simulink subsystem "Driver_Input"  (R2021b)
settings: Solver=VariableStepAuto  StartTime=0.0  StopTime=10.0  RelTol=1e-3
PostLoadFcn:
  | if any(exist('dsrtsu_mdlpostloadfcn', 'file') ~= 0), dsrtsu_mdlpostloadfcn('Execute', bdroot); end
libraries: simulink x9, dspstat3 x7, rtican x3, rti1401lib_adc_type4 x1
(part 2 of 2)

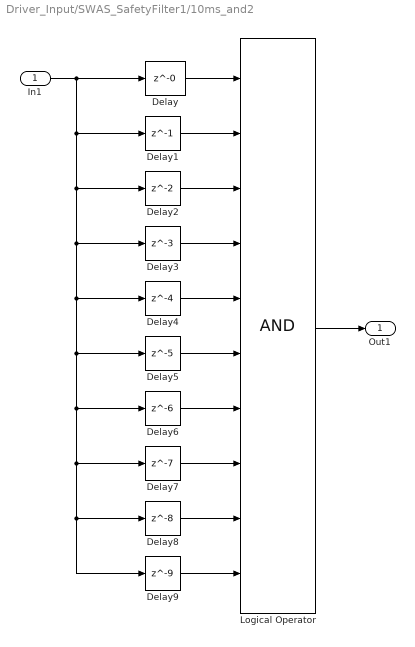
== system Driver_Input/SWAS_SafetyFilter1/10ms_and2 ==
  In1 : Inport
  Delay : Delay  DelayLength=0  InitialCondition=0
  Delay1 : Delay  DelayLength=1  InitialCondition=0
  Delay2 : Delay  InitialCondition=0
  Delay3 : Delay  DelayLength=3  InitialCondition=0
  Delay4 : Delay  DelayLength=4  InitialCondition=0
  Delay5 : Delay  DelayLength=5  InitialCondition=0
  Delay6 : Delay  DelayLength=6  InitialCondition=0
  Delay7 : Delay  DelayLength=7  InitialCondition=0
  Delay8 : Delay  DelayLength=8  InitialCondition=0
  Delay9 : Delay  DelayLength=9  InitialCondition=0
  Logical Operator : Logic  Inputs=10  AllPortsSameDT=off  OutDataTypeStr=boolean
  Out1 : Outport  VectorParamsAs1DForOutWhenUnconnected=off
  wires:
  Delay2/1 -> Logical Operator/3
  Delay8/1 -> Logical Operator/9
  In1/1 -> Delay9/1, Delay8/1, Delay7/1, Delay6/1, Delay5/1, Delay4/1, Delay3/1, Delay2/1, Delay1/1, Delay/1
  Delay/1 -> Logical Operator/1
  Delay1/1 -> Logical Operator/2
  Delay3/1 -> Logical Operator/4
  Delay4/1 -> Logical Operator/5
  Delay9/1 -> Logical Operator/10
  Delay5/1 -> Logical Operator/6
  Delay7/1 -> Logical Operator/8
  Delay6/1 -> Logical Operator/7
  Logical Operator/1 -> Out1/1

== matlab function Driver_Input/Calibration5/MATLAB Function ==
  data: mV input; bar output
function bar = fcn(mV)

bar = 10/4000*(mV-500)*10;

== matlab function Driver_Input/Calibration6/MATLAB Function ==
  data: mV input; bar output
function bar = fcn(mV)

bar = 10/4000*(mV-500)*10;
